simulink model "coursework2model2"  (R2024b)
settings: Solver=VariableStepAuto  StartTime=0.0  StopTime=10  RelTol=1e-3
undefined symbols (not defined in the file): K, rho
settings Model: Creator=user  LastModifiedBy=Oteng_fy0f5z9
settings RTWCC: GPUComputeCapability=3.5

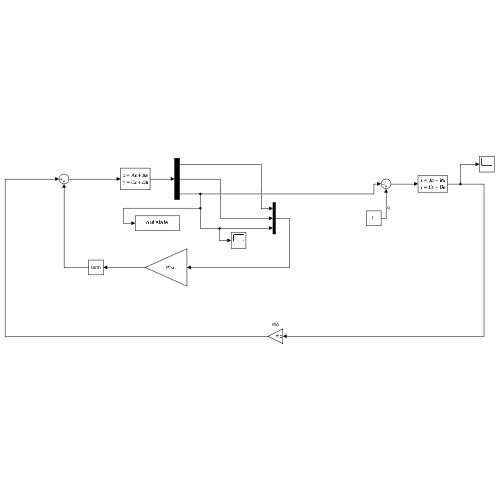
[thumbnail: Simulink's stored preview of the top-level diagram]
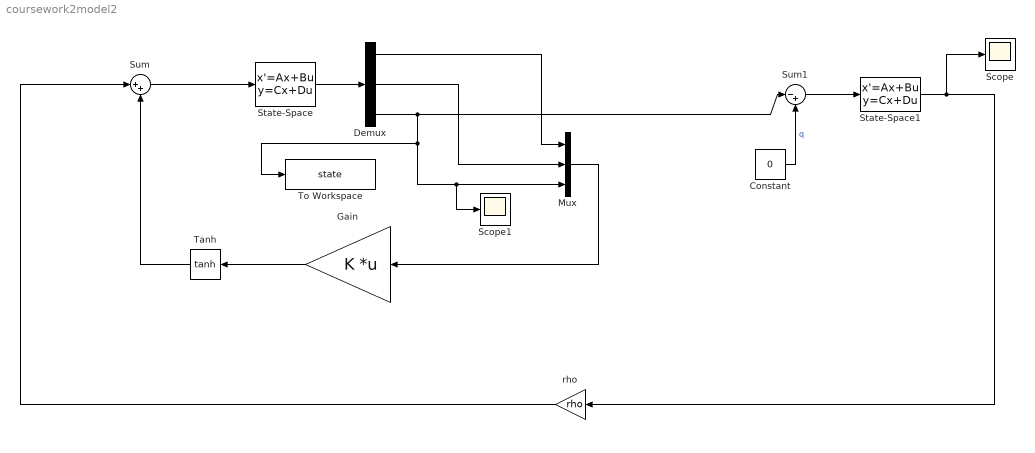
== system coursework2model2 ==
  Constant : Constant  Value=0
  Demux : Demux  Outputs=3
  Gain : Gain  Gain=K  Multiplication=Matrix(K*u)
  Mux : Mux  Inputs=3
  Scope : Scope
  Scope1 : Scope
  State-Space : StateSpace  A=[-10 -0 10;0 -100 100;0 0 -1]  B=[0;0;1]  C=[1 0 0;0 1 0; 0 0 1]  D=[0;0;0]  InitialCondition=[0,0,0.2]  ParameterTunability=Unconstrained
  State-Space1 : StateSpace  A=[0 1; -2000 -100]  B=[0;1000]  C=[30 1]  D=0  InitialCondition=0
  Sum : Sum  Inputs=|++
  Sum1 : Sum  Inputs=|-+
  Tanh : Trigonometry  Operator=tanh
  To Workspace : ToWorkspace  VariableName=state  SaveFormat=Timeseries  SampleTime=-1
  rho : Gain  Gain=rho
  wires:
  Mux/1 -> Gain/1
  Tanh/1 -> Sum/2
  Gain/1 -> Tanh/1
  Sum/1 -> State-Space/1
  State-Space/1 -> Demux/1
  rho/1 -> Sum/1
  Sum1/1 -> State-Space1/1
  State-Space1/1 -> Scope/1, rho/1
  Constant/1 -> Sum1/2  "q"
  Demux/1 -> Mux/1
  Demux/2 -> Mux/2
  Demux/3 -> Scope1/1, Mux/3, To Workspace/1, Sum1/1
